simulink model "TD_ex7"  (Simulink 9.1)
settings: Solver=ode45  StartTime=0.0  StopTime=10.0  RelTol=1e-3  EnableMultiTasking=on
libraries: cstblocks x4
settings Model: SuppressorTable=22 serialization::archive 11 0 6 0 0 0 0 0  Creator=Mokrane  LastModifiedBy=Mokrane
settings DataIOCC: LimitDataPoints=on  SignalLoggingSaveFormat=ModelDataLogs  SignalLoggingName=sigsOut
settings OptimizationCC: LifeSpan=auto
settings DebuggingCC: SaveWithParameterizedLinksMsg=none  SignalResolutionControl=TryResolveAllWithWarning  MultiTaskDSMMsg=warning  MultiTaskCondExecSysMsg=none  SFUnexpectedBacktrackingDiag=error  SFNoUnconditionalDefaultTransitionDiag=error  SFExecutionAtInitializationDiag=warning
settings HardwareCC: TargetUnknown=on
settings CodeAppCC: StateflowObjectComments=off

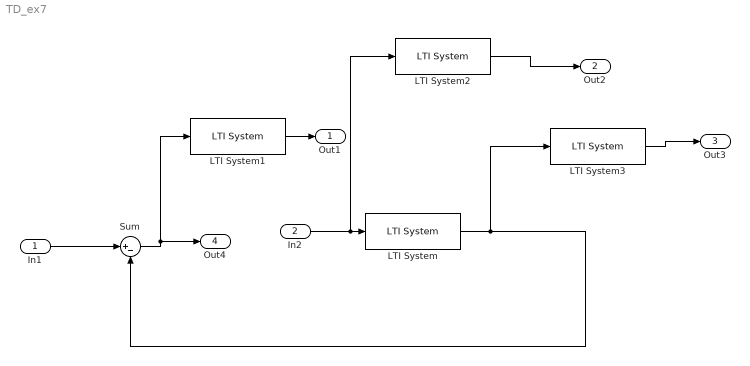
== system TD_ex7 ==
  In1 : Inport
  In2 : Inport  Port=2
  LTI System : cstblocks/LTI System  sys=Gn  IC=[]
  LTI System1 : cstblocks/LTI System  sys=W1  IC=[]
  LTI System2 : cstblocks/LTI System  sys=W2  IC=[]
  LTI System3 : cstblocks/LTI System  sys=W3  IC=[]
  Sum : Sum  Inputs=|+-  SaturateOnIntegerOverflow=on
  Out1 : Outport
  Out2 : Outport  Port=2
  Out3 : Outport  Port=3
  Out4 : Outport  Port=4
  wires:
  LTI System/1 -> Sum/2, LTI System3/1
  Sum/1 -> LTI System1/1, Out4/1
  LTI System1/1 -> Out1/1
  In1/1 -> Sum/1
  In2/1 -> LTI System/1, LTI System2/1
  LTI System2/1 -> Out2/1
  LTI System3/1 -> Out3/1
